simulink model "QuadRotor_PID_Simulink3d"  (R2014a)
settings: Solver=ode45  StartTime=0.0  StopTime=inf
PreLoadFcn:
  | load CommandsBus
model workspace (MAT data in the model file):
  MCOS : class17 (value not decoded)
  MCOS : class17 (value not decoded)
undefined symbols (not defined in the file or in its folder): X, Y, Z
libraries: sm_lib x829, nesl_utility x156, simulink x12, fl_lib x4, vrlib x4, aerolibtransform2 x1
(part 18 of 18)

== system QuadRotor_PID_Simulink3d/quadSimulation/Plant_Quad_Base/Quad_Yaw_Altitude/QuadRotor/P4/MotorD/Helice_1_RIGID ==
  ReferenceFrame : sm_lib/Frames and Transforms/Reference Frame  BlockFunction=simmechanics.library.frames_transforms.reference_frame
  Solid : sm_lib/Body Elements/Solid  InertiaType=Custom  Mass=0.00049709299999999999  MassUnits=kg  CenterOfMass=[0 0 -0.00012752400000000001]  CenterOfMassUnits=mm  MomentsOfInertia=[0.0011848399999999999 0.31476899999999997 0.31557499999999999]  MomentsOfInertiaUnits=kg*mm^2  ProductsOfInertia=[0 0 -7.1669699999999998e-06]  ProductsOfInertiaUnits=kg*mm^2  DensityBased=on  Density=1000  DensityUnits=kg/(m^3)  GraphicType=FromGeometry  MarkerShape=Sphere  MarkerSize=10  MarkerSizeUnits=m  GraphicVisPropType=SimpleVisualProperties  GraphicDiffuseColor=[1 1 1]  GraphicSpecularColor=[0.5 0.5 0.5 1.0]  GraphicAmbientColor=[0.15 0.15 0.15 1.0]  GraphicEmissiveColor=[0.0 0.0 0.0 1.0]  GraphicShininess=75  GraphicOpacity=1  GeometryShape=FromFile  RectangleSize=[1 1]  RectangleSizeUnits=m  BrickDimensions=[1 1 1]  BrickDimensionUnits=m  CylinderRadius=1  CylinderRadiusUnits=m  CylinderLength=1  CylinderLengthUnits=m  SphereRadius=1  SphereRadiusUnits=m  EllipsoidRadii=[1 1 1]  EllipsoidRadiiUnits=m  ExtrusionCrossSection=[1 1; -1 1; -1 -1; 1 -1]  ExtrusionCrossSectionUnits=m  ExtrusionLength=1  ExtrusionLengthUnits=m  PolygonNumSides=3  PolygonOuterRadius=1  PolygonOuterRadiusUnits=m  ExtGeomFileType=STL  ExtGeomFileName=Helice_Valor predeterminado_sldprt.STL  ExtGeomFileUnits=mm  RevolutionCrossSection=[1 1; 1 -1; 2 -1; 2 1]  RevolutionCrossSectionUnits=m  RevolutionExtent=Full  RevolutionAngle=180  RevolutionAngleUnits=deg  BlockFunction=simmechanics.library.body_elements.solid
  F : PMIOPort  Port=1  Side=Left
  connections:
  Solid/RConn1 -- ReferenceFrame/RConn1 -- F/RConn1

== system QuadRotor_PID_Simulink3d/quadSimulation/Plant_Quad_Base/Quad_Yaw_Altitude/QuadRotor/P4/MotorD/x18_11_2000kv_Micro_Brushless_1_RIGID ==
  ReferenceFrame : sm_lib/Frames and Transforms/Reference Frame  BlockFunction=simmechanics.library.frames_transforms.reference_frame
  Solid : sm_lib/Body Elements/Solid  InertiaType=Custom  Mass=10  MassUnits=g  CenterOfMass=[0 12.8438 0]  CenterOfMassUnits=mm  MomentsOfInertia=[0.43731300000000001 0.28562900000000002 0.43731300000000001]  MomentsOfInertiaUnits=kg*mm^2  ProductsOfInertia=[0 0 0]  ProductsOfInertiaUnits=kg*mm^2  DensityBased=on  Density=1000  DensityUnits=kg/(m^3)  GraphicType=FromGeometry  MarkerShape=Sphere  MarkerSize=10  MarkerSizeUnits=m  GraphicVisPropType=SimpleVisualProperties  GraphicDiffuseColor=[0.894118 0.913725 0.929412]  GraphicSpecularColor=[0.5 0.5 0.5 1.0]  GraphicAmbientColor=[0.15 0.15 0.15 1.0]  GraphicEmissiveColor=[0.0 0.0 0.0 1.0]  GraphicShininess=75  GraphicOpacity=1  GeometryShape=FromFile  RectangleSize=[1 1]  RectangleSizeUnits=m  BrickDimensions=[1 1 1]  BrickDimensionUnits=m  CylinderRadius=1  CylinderRadiusUnits=m  CylinderLength=1  CylinderLengthUnits=m  SphereRadius=1  SphereRadiusUnits=m  EllipsoidRadii=[1 1 1]  EllipsoidRadiiUnits=m  ExtrusionCrossSection=[1 1; -1 1; -1 -1; 1 -1]  ExtrusionCrossSectionUnits=m  ExtrusionLength=1  ExtrusionLengthUnits=m  PolygonNumSides=3  PolygonOuterRadius=1  PolygonOuterRadiusUnits=m  ExtGeomFileType=STL  ExtGeomFileName=18-11 2000kv Micro Brushless_Valor predeterminado_sldprt.STL  ExtGeomFileUnits=mm  RevolutionCrossSection=[1 1; 1 -1; 2 -1; 2 1]  RevolutionCrossSectionUnits=m  RevolutionExtent=Full  RevolutionAngle=180  RevolutionAngleUnits=deg  BlockFunction=simmechanics.library.body_elements.solid
  F : PMIOPort  Port=1  Side=Left
  connections:
  Solid/RConn1 -- ReferenceFrame/RConn1 -- F/RConn1

== matlab function QuadRotor_PID_Simulink3d/quadSimulation/Plant_Quad_Base/Quad_Roll_Pitch_Yaw_Altitude/QuadRotor/P2/MotorA/Thrust ==
  data: revSpeed input; Thrust output; revCnst input; revTqCnst input; Torque output
function [Thrust, Torque]  = generateThrust(revSpeed, revCnst, revTqCnst)
%#codegen
Torque = revSpeed * revTqCnst;

% Always give positive thrust (Point up)
Thrust = revCnst * revSpeed;
if (Thrust < 0)
   Thrust = Thrust * -1; 
end

== matlab function QuadRotor_PID_Simulink3d/quadSimulation/Plant_Quad_Base/Quad_Roll_Pitch_Yaw_Altitude/QuadRotor/P3/MotorC/Thrust ==
  data: revSpeed input; Thrust output; revCnst input; revTqCnst input; Torque output
function [Thrust, Torque]  = generateThrust(revSpeed, revCnst, revTqCnst)
%#codegen
Torque = revSpeed * revTqCnst;

% Always give positive thrust (Point up)
Thrust = revCnst * revSpeed;
if (Thrust < 0)
   Thrust = Thrust * -1; 
end

== matlab function QuadRotor_PID_Simulink3d/quadSimulation/Plant_Quad_Base/Quad_Roll_Pitch_Yaw_Altitude/QuadRotor/P4/MotorD/Thrust ==
  data: revSpeed input; Thrust output; revCnst input; revTqCnst input; Torque output
function [Thrust, Torque]  = generateThrust(revSpeed, revCnst, revTqCnst)
%#codegen
Torque = revSpeed * revTqCnst;

% Always give positive thrust (Point up)
Thrust = revCnst * revSpeed;
if (Thrust < 0)
   Thrust = Thrust * -1; 
end

== matlab function QuadRotor_PID_Simulink3d/quadSimulation/Plant_Quad_Base/Quad_Roll_Pitch_Yaw_Altitude/Convert/ConvertAngle ==
  data: radAngle input; AngleDeg output
function AngleDeg = getAngleDeg(radAngle)
%#codegen
AngleDeg = 0;
angleAcc = radAngle / pi;

AngleDeg = radAngle * (180/pi);
if abs(AngleDeg) > 360
    AngleDeg = mod(AngleDeg,360);
end

== matlab function QuadRotor_PID_Simulink3d/quadSimulation/Plant_Quad_Base/Quad_Roll_Pitch_Yaw_Altitude/Convert1/ConvertAngle ==
  data: radAngle input; AngleDeg output
function AngleDeg = getAngleDeg(radAngle)
%#codegen
AngleDeg = 0;
angleAcc = radAngle / pi;

AngleDeg = radAngle * (180/pi);
if abs(AngleDeg) > 360
    AngleDeg = mod(AngleDeg,360);
end

== matlab function QuadRotor_PID_Simulink3d/quadSimulation/Plant_Quad_Base/Quad_Roll_Pitch_Yaw_Altitude/Convert2/ConvertAngle ==
  data: radAngle input; AngleDeg output
function AngleDeg = getAngleDeg(radAngle)
%#codegen
AngleDeg = 0;
angleAcc = radAngle / pi;

AngleDeg = radAngle * (180/pi);
if abs(AngleDeg) > 360
    AngleDeg = mod(AngleDeg,360);
end
%AngleDeg = angleAcc * (180/pi);

== matlab function QuadRotor_PID_Simulink3d/quadSimulation/Controller/SaturateRollCmd ==
  data: spdRef input; spdOut output; inSpd input; maxVar input
function spdOut = fcn(spdRef, inSpd, maxVar)
%#codegen
minLim = -(spdRef * (maxVar/100));
maxLim = (spdRef * (maxVar/100));

spdOut = inSpd;

if inSpd > maxLim
   spdOut = maxLim;
   return;
elseif inSpd < minLim    
   spdOut = minLim; 
   return;
end

end

== matlab function QuadRotor_PID_Simulink3d/quadSimulation/Controller/SaturatePitchCmd ==
  data: spdRef input; spdOut output; inSpd input; maxVar input
function spdOut = fcn(spdRef, inSpd, maxVar)
%#codegen
minLim = -(spdRef * (maxVar/100));
maxLim = (spdRef * (maxVar/100));

spdOut = inSpd;

if inSpd > maxLim
   spdOut = maxLim;
   return;
elseif inSpd < minLim    
   spdOut = minLim; 
   return;
end

end

== matlab function QuadRotor_PID_Simulink3d/quadSimulation/Controller/SaturateRollCmd1 ==
  data: spdRef input; spdOut output; inSpd input; maxVar input
function spdOut = fcn(spdRef, inSpd, maxVar)
%#codegen
%minLim = spdRef - (spdRef * (maxVar/100));
%maxLim = spdRef + (spdRef * (maxVar/100));
minLim = -(spdRef * (maxVar/100));
maxLim = (spdRef * (maxVar/100));

spdOut = inSpd;

if inSpd > maxLim
   spdOut = maxLim;
   return;
elseif inSpd < minLim    
   spdOut = minLim; 
   return;
end

end

== matlab function QuadRotor_PID_Simulink3d/quadSimulation/Plant_Quad_Base/Quad_Altitude/Convert/ConvertAngle ==
  data: radAngle input; AngleDeg output
function AngleDeg = getAngleDeg(radAngle)
%#codegen
AngleDeg = 0;
angleAcc = radAngle / pi;

AngleDeg = radAngle * (180/pi);
if abs(AngleDeg) > 360
    AngleDeg = mod(AngleDeg,360);
end

== matlab function QuadRotor_PID_Simulink3d/quadSimulation/Plant_Quad_Base/Quad_Altitude/Convert1/ConvertAngle ==
  data: radAngle input; AngleDeg output
function AngleDeg = getAngleDeg(radAngle)
%#codegen

AngleDeg = radAngle * (180/pi);
if abs(AngleDeg) > 360
    AngleDeg = mod(AngleDeg,360);
end

== matlab function QuadRotor_PID_Simulink3d/quadSimulation/Plant_Quad_Base/Quad_Altitude/Convert2/ConvertAngle ==
  data: radAngle input; AngleDeg output
function AngleDeg = getAngleDeg(radAngle)
%#codegen
AngleDeg = 0;
angleAcc = radAngle / pi;

AngleDeg = radAngle * (180/pi);
if abs(AngleDeg) > 360
    AngleDeg = mod(AngleDeg,360);
end
%AngleDeg = angleAcc * (180/pi);

== matlab function QuadRotor_PID_Simulink3d/quadSimulation/Plant_Quad_Base/Quad_Altitude/QuadRotor/P1/MotorB/Thrust ==
  data: revSpeed input; Thrust output; revCnst input; revTqCnst input; Torque output
function [Thrust, Torque]  = generateThrust(revSpeed, revCnst, revTqCnst)
%#codegen
Torque = revSpeed * revTqCnst;

% Always give positive thrust (Point up)
Thrust = abs(revCnst * revSpeed);

== matlab function QuadRotor_PID_Simulink3d/quadSimulation/Plant_Quad_Base/Quad_Altitude/QuadRotor/P2/MotorA/Thrust ==
  data: revSpeed input; Thrust output; revCnst input; revTqCnst input; Torque output
function [Thrust, Torque]  = generateThrust(revSpeed, revCnst, revTqCnst)
%#codegen
Torque = revSpeed * revTqCnst;

% Always give positive thrust (Point up)
Thrust = revCnst * revSpeed;
if (Thrust < 0)
   Thrust = Thrust * -1; 
end

== matlab function QuadRotor_PID_Simulink3d/quadSimulation/Plant_Quad_Base/Quad_Altitude/QuadRotor/P3/MotorC/Thrust ==
  data: revSpeed input; Thrust output; revCnst input; revTqCnst input; Torque output
function [Thrust, Torque]  = generateThrust(revSpeed, revCnst, revTqCnst)
%#codegen
Torque = revSpeed * revTqCnst;

% Always give positive thrust (Point up)
Thrust = revCnst * revSpeed;
if (Thrust < 0)
   Thrust = Thrust * -1; 
end

== matlab function QuadRotor_PID_Simulink3d/quadSimulation/Plant_Quad_Base/Quad_Altitude/QuadRotor/P4/MotorD/Thrust ==
  data: revSpeed input; Thrust output; revCnst input; revTqCnst input; Torque output
function [Thrust, Torque]  = generateThrust(revSpeed, revCnst, revTqCnst)
%#codegen
Torque = revSpeed * revTqCnst;

% Always give positive thrust (Point up)
Thrust = revCnst * revSpeed;
if (Thrust < 0)
   Thrust = Thrust * -1; 
end

== matlab function QuadRotor_PID_Simulink3d/quadSimulation/Plant_Quad_Base/Quad_Pitch/Convert/ConvertAngle ==
  data: radAngle input; AngleDeg output
function AngleDeg = getAngleDeg(radAngle)
%#codegen
AngleDeg = 0;
angleAcc = radAngle / pi;

AngleDeg = radAngle * (180/pi);
if abs(AngleDeg) > 360
    AngleDeg = mod(AngleDeg,360);
end

== matlab function QuadRotor_PID_Simulink3d/quadSimulation/Plant_Quad_Base/Quad_Pitch/Convert1/ConvertAngle ==
  data: radAngle input; AngleDeg output
function AngleDeg = getAngleDeg(radAngle)
%#codegen
AngleDeg = 0;
angleAcc = radAngle / pi;

AngleDeg = radAngle * (180/pi);
if abs(AngleDeg) > 360
    AngleDeg = mod(AngleDeg,360);
end

== matlab function QuadRotor_PID_Simulink3d/quadSimulation/Plant_Quad_Base/Quad_Pitch/Convert2/ConvertAngle ==
  data: radAngle input; AngleDeg output
function AngleDeg = getAngleDeg(radAngle)
%#codegen
AngleDeg = 0;
angleAcc = radAngle / pi;

AngleDeg = radAngle * (180/pi);
if abs(AngleDeg) > 360
    AngleDeg = mod(AngleDeg,360);
end
%AngleDeg = angleAcc * (180/pi);

== matlab function QuadRotor_PID_Simulink3d/quadSimulation/Plant_Quad_Base/Quad_Pitch/QuadRotor/P1/MotorB/Thrust ==
  data: revSpeed input; Thrust output; revCnst input; revTqCnst input; Torque output
function [Thrust, Torque]  = generateThrust(revSpeed, revCnst, revTqCnst)
%#codegen
Torque = revSpeed * revTqCnst;

% Always give positive thrust (Point up)
Thrust = abs(revCnst * revSpeed);

== matlab function QuadRotor_PID_Simulink3d/quadSimulation/Plant_Quad_Base/Quad_Pitch/QuadRotor/P2/MotorA/Thrust ==
  data: revSpeed input; Thrust output; revCnst input; revTqCnst input; Torque output
function [Thrust, Torque]  = generateThrust(revSpeed, revCnst, revTqCnst)
%#codegen
Torque = revSpeed * revTqCnst;

% Always give positive thrust (Point up)
Thrust = revCnst * revSpeed;
if (Thrust < 0)
   Thrust = Thrust * -1; 
end

== matlab function QuadRotor_PID_Simulink3d/quadSimulation/Plant_Quad_Base/Quad_Pitch/QuadRotor/P3/MotorC/Thrust ==
  data: revSpeed input; Thrust output; revCnst input; revTqCnst input; Torque output
function [Thrust, Torque]  = generateThrust(revSpeed, revCnst, revTqCnst)
%#codegen
Torque = revSpeed * revTqCnst;

% Always give positive thrust (Point up)
Thrust = revCnst * revSpeed;
if (Thrust < 0)
   Thrust = Thrust * -1; 
end

== matlab function QuadRotor_PID_Simulink3d/quadSimulation/Plant_Quad_Base/Quad_Pitch/QuadRotor/P4/MotorD/Thrust ==
  data: revSpeed input; Thrust output; revCnst input; revTqCnst input; Torque output
function [Thrust, Torque]  = generateThrust(revSpeed, revCnst, revTqCnst)
%#codegen
Torque = revSpeed * revTqCnst;

% Always give positive thrust (Point up)
Thrust = revCnst * revSpeed;
if (Thrust < 0)
   Thrust = Thrust * -1; 
end

== matlab function QuadRotor_PID_Simulink3d/quadSimulation/Plant_Quad_Base/Quad_Yaw/Convert/ConvertAngle ==
  data: radAngle input; AngleDeg output
function AngleDeg = getAngleDeg(radAngle)
%#codegen
AngleDeg = 0;
angleAcc = radAngle / pi;

AngleDeg = radAngle * (180/pi);
if abs(AngleDeg) > 360
    AngleDeg = mod(AngleDeg,360);
end

== matlab function QuadRotor_PID_Simulink3d/quadSimulation/Plant_Quad_Base/Quad_Yaw/Convert1/ConvertAngle ==
  data: radAngle input; AngleDeg output
function AngleDeg = getAngleDeg(radAngle)
%#codegen
AngleDeg = 0;
angleAcc = radAngle / pi;

AngleDeg = radAngle * (180/pi);
if abs(AngleDeg) > 360
    AngleDeg = mod(AngleDeg,360);
end

== matlab function QuadRotor_PID_Simulink3d/quadSimulation/Plant_Quad_Base/Quad_Yaw/Convert2/ConvertAngle ==
  data: radAngle input; AngleDeg output
function AngleDeg = getAngleDeg(radAngle)
%#codegen
AngleDeg = 0;
angleAcc = radAngle / pi;

AngleDeg = radAngle * (180/pi);
if abs(AngleDeg) > 360
    AngleDeg = mod(AngleDeg,360);
end
%AngleDeg = angleAcc * (180/pi);

== matlab function QuadRotor_PID_Simulink3d/quadSimulation/Plant_Quad_Base/Quad_Yaw/QuadRotor/P1/MotorB/Thrust ==
  data: revSpeed input; Thrust output; revCnst input; revTqCnst input; Torque output
function [Thrust, Torque]  = generateThrust(revSpeed, revCnst, revTqCnst)
%#codegen
Torque = revSpeed * revTqCnst;

% Always give positive thrust (Point up)
Thrust = abs(revCnst * revSpeed);

== matlab function QuadRotor_PID_Simulink3d/quadSimulation/Plant_Quad_Base/Quad_Yaw/QuadRotor/P2/MotorA/Thrust ==
  data: revSpeed input; Thrust output; revCnst input; revTqCnst input; Torque output
function [Thrust, Torque]  = generateThrust(revSpeed, revCnst, revTqCnst)
%#codegen
Torque = revSpeed * revTqCnst;

% Always give positive thrust (Point up)
Thrust = revCnst * revSpeed;
if (Thrust < 0)
   Thrust = Thrust * -1; 
end

== matlab function QuadRotor_PID_Simulink3d/quadSimulation/Plant_Quad_Base/Quad_Yaw/QuadRotor/P3/MotorC/Thrust ==
  data: revSpeed input; Thrust output; revCnst input; revTqCnst input; Torque output
function [Thrust, Torque]  = generateThrust(revSpeed, revCnst, revTqCnst)
%#codegen
Torque = revSpeed * revTqCnst;

% Always give positive thrust (Point up)
Thrust = revCnst * revSpeed;
if (Thrust < 0)
   Thrust = Thrust * -1; 
end

== matlab function QuadRotor_PID_Simulink3d/quadSimulation/Plant_Quad_Base/Quad_Yaw/QuadRotor/P4/MotorD/Thrust ==
  data: revSpeed input; Thrust output; revCnst input; revTqCnst input; Torque output
function [Thrust, Torque]  = generateThrust(revSpeed, revCnst, revTqCnst)
%#codegen
Torque = revSpeed * revTqCnst;

% Always give positive thrust (Point up)
Thrust = revCnst * revSpeed;
if (Thrust < 0)
   Thrust = Thrust * -1; 
end

== matlab function QuadRotor_PID_Simulink3d/quadSimulation/Plant_Quad_Base/Quad_Roll/Convert/ConvertAngle ==
  data: radAngle input; AngleDeg output
function AngleDeg = getAngleDeg(radAngle)
%#codegen
AngleDeg = 0;
angleAcc = radAngle / pi;

AngleDeg = radAngle * (180/pi);
if abs(AngleDeg) > 360
    AngleDeg = mod(AngleDeg,360);
end

== matlab function QuadRotor_PID_Simulink3d/quadSimulation/Plant_Quad_Base/Quad_Roll/Convert1/ConvertAngle ==
  data: radAngle input; AngleDeg output
function AngleDeg = getAngleDeg(radAngle)
%#codegen
AngleDeg = 0;
angleAcc = radAngle / pi;

AngleDeg = radAngle * (180/pi);
if abs(AngleDeg) > 360
    AngleDeg = mod(AngleDeg,360);
end

== matlab function QuadRotor_PID_Simulink3d/quadSimulation/Plant_Quad_Base/Quad_Roll/Convert2/ConvertAngle ==
  data: radAngle input; AngleDeg output
function AngleDeg = getAngleDeg(radAngle)
%#codegen
AngleDeg = 0;
angleAcc = radAngle / pi;

AngleDeg = radAngle * (180/pi);
if abs(AngleDeg) > 360
    AngleDeg = mod(AngleDeg,360);
end
%AngleDeg = angleAcc * (180/pi);

== matlab function QuadRotor_PID_Simulink3d/quadSimulation/Plant_Quad_Base/Quad_Roll/QuadRotor/P1/MotorB/Thrust ==
  data: revSpeed input; Thrust output; revCnst input; revTqCnst input; Torque output
function [Thrust, Torque]  = generateThrust(revSpeed, revCnst, revTqCnst)
%#codegen
Torque = revSpeed * revTqCnst;

% Always give positive thrust (Point up)
Thrust = abs(revCnst * revSpeed);

== matlab function QuadRotor_PID_Simulink3d/quadSimulation/Plant_Quad_Base/Quad_Roll/QuadRotor/P2/MotorA/Thrust ==
  data: revSpeed input; Thrust output; revCnst input; revTqCnst input; Torque output
function [Thrust, Torque]  = generateThrust(revSpeed, revCnst, revTqCnst)
%#codegen
Torque = revSpeed * revTqCnst;

% Always give positive thrust (Point up)
Thrust = revCnst * revSpeed;
if (Thrust < 0)
   Thrust = Thrust * -1; 
end

== matlab function QuadRotor_PID_Simulink3d/quadSimulation/Plant_Quad_Base/Quad_Roll_Pitch_Yaw_Altitude/QuadRotor/P1/MotorB/Thrust ==
  data: revSpeed input; Thrust output; revCnst input; revTqCnst input; Torque output
function [Thrust, Torque]  = generateThrust(revSpeed, revCnst, revTqCnst)
%#codegen
Torque = revSpeed * revTqCnst;

% Always give positive thrust (Point up)
Thrust = abs(revCnst * revSpeed);

== matlab function QuadRotor_PID_Simulink3d/quadSimulation/Plant_Quad_Base/Quad_Roll/QuadRotor/P3/MotorC/Thrust ==
  data: revSpeed input; Thrust output; revCnst input; revTqCnst input; Torque output
function [Thrust, Torque]  = generateThrust(revSpeed, revCnst, revTqCnst)
%#codegen
Torque = revSpeed * revTqCnst;

% Always give positive thrust (Point up)
Thrust = revCnst * revSpeed;
if (Thrust < 0)
   Thrust = Thrust * -1; 
end

== matlab function QuadRotor_PID_Simulink3d/quadSimulation/Plant_Quad_Base/Quad_Roll/QuadRotor/P4/MotorD/Thrust ==
  data: revSpeed input; Thrust output; revCnst input; revTqCnst input; Torque output
function [Thrust, Torque]  = generateThrust(revSpeed, revCnst, revTqCnst)
%#codegen
Torque = revSpeed * revTqCnst;

% Always give positive thrust (Point up)
Thrust = revCnst * revSpeed;
if (Thrust < 0)
   Thrust = Thrust * -1; 
end

== matlab function QuadRotor_PID_Simulink3d/quadSimulation/Plant_Quad_Base/Quad_Roll_Pitch_Yaw/Convert/ConvertAngle ==
  data: radAngle input; AngleDeg output
function AngleDeg = getAngleDeg(radAngle)
%#codegen
AngleDeg = 0;
angleAcc = radAngle / pi;

AngleDeg = radAngle * (180/pi);
if abs(AngleDeg) > 360
    AngleDeg = mod(AngleDeg,360);
end

== matlab function QuadRotor_PID_Simulink3d/quadSimulation/Plant_Quad_Base/Quad_Roll_Pitch_Yaw/Convert1/ConvertAngle ==
  data: radAngle input; AngleDeg output
function AngleDeg = getAngleDeg(radAngle)
%#codegen
AngleDeg = 0;
angleAcc = radAngle / pi;

AngleDeg = radAngle * (180/pi);
if abs(AngleDeg) > 360
    AngleDeg = mod(AngleDeg,360);
end

== matlab function QuadRotor_PID_Simulink3d/quadSimulation/Plant_Quad_Base/Quad_Roll_Pitch_Yaw/Convert2/ConvertAngle ==
  data: radAngle input; AngleDeg output
function AngleDeg = getAngleDeg(radAngle)
%#codegen
AngleDeg = 0;
angleAcc = radAngle / pi;

AngleDeg = radAngle * (180/pi);
if abs(AngleDeg) > 360
    AngleDeg = mod(AngleDeg,360);
end
%AngleDeg = angleAcc * (180/pi);

== matlab function QuadRotor_PID_Simulink3d/quadSimulation/Plant_Quad_Base/Quad_Roll_Pitch_Yaw/QuadRotor/P1/MotorB/Thrust ==
  data: revSpeed input; Thrust output; revCnst input; revTqCnst input; Torque output
function [Thrust, Torque]  = generateThrust(revSpeed, revCnst, revTqCnst)
%#codegen
Torque = revSpeed * revTqCnst;

% Always give positive thrust (Point up)
Thrust = abs(revCnst * revSpeed);

== matlab function QuadRotor_PID_Simulink3d/quadSimulation/Plant_Quad_Base/Quad_Roll_Pitch_Yaw/QuadRotor/P2/MotorA/Thrust ==
  data: revSpeed input; Thrust output; revCnst input; revTqCnst input; Torque output
function [Thrust, Torque]  = generateThrust(revSpeed, revCnst, revTqCnst)
%#codegen
Torque = revSpeed * revTqCnst;

% Always give positive thrust (Point up)
Thrust = revCnst * revSpeed;
if (Thrust < 0)
   Thrust = Thrust * -1; 
end

== matlab function QuadRotor_PID_Simulink3d/quadSimulation/Plant_Quad_Base/Quad_Roll_Pitch_Yaw/QuadRotor/P3/MotorC/Thrust ==
  data: revSpeed input; Thrust output; revCnst input; revTqCnst input; Torque output
function [Thrust, Torque]  = generateThrust(revSpeed, revCnst, revTqCnst)
%#codegen
Torque = revSpeed * revTqCnst;

% Always give positive thrust (Point up)
Thrust = revCnst * revSpeed;
if (Thrust < 0)
   Thrust = Thrust * -1; 
end

== matlab function QuadRotor_PID_Simulink3d/quadSimulation/Plant_Quad_Base/Quad_Roll_Pitch_Yaw/QuadRotor/P4/MotorD/Thrust ==
  data: revSpeed input; Thrust output; revCnst input; revTqCnst input; Torque output
function [Thrust, Torque]  = generateThrust(revSpeed, revCnst, revTqCnst)
%#codegen
Torque = revSpeed * revTqCnst;

% Always give positive thrust (Point up)
Thrust = revCnst * revSpeed;
if (Thrust < 0)
   Thrust = Thrust * -1; 
end

== matlab function QuadRotor_PID_Simulink3d/quadSimulation/Plant_Quad_Base/Quad_Yaw_Altitude/Convert/ConvertAngle ==
  data: radAngle input; AngleDeg output
function AngleDeg = getAngleDeg(radAngle)
%#codegen
AngleDeg = 0;
angleAcc = radAngle / pi;

AngleDeg = radAngle * (180/pi);
if abs(AngleDeg) > 360
    AngleDeg = mod(AngleDeg,360);
end

== matlab function QuadRotor_PID_Simulink3d/quadSimulation/Plant_Quad_Base/Quad_Yaw_Altitude/Convert1/ConvertAngle ==
  data: radAngle input; AngleDeg output
function AngleDeg = getAngleDeg(radAngle)
%#codegen
AngleDeg = 0;
angleAcc = radAngle / pi;

AngleDeg = radAngle * (180/pi);
if abs(AngleDeg) > 360
    AngleDeg = mod(AngleDeg,360);
end

== matlab function QuadRotor_PID_Simulink3d/quadSimulation/Plant_Quad_Base/Quad_Yaw_Altitude/Convert2/ConvertAngle ==
  data: radAngle input; AngleDeg output
function AngleDeg = getAngleDeg(radAngle)
%#codegen
AngleDeg = 0;
angleAcc = radAngle / pi;

AngleDeg = radAngle * (180/pi);
if abs(AngleDeg) > 360
    AngleDeg = mod(AngleDeg,360);
end
%AngleDeg = angleAcc * (180/pi);

== matlab function QuadRotor_PID_Simulink3d/quadSimulation/Plant_Quad_Base/Quad_Yaw_Altitude/QuadRotor/P1/MotorB/Thrust ==
  data: revSpeed input; Thrust output; revCnst input; revTqCnst input; Torque output
function [Thrust, Torque]  = generateThrust(revSpeed, revCnst, revTqCnst)
%#codegen
Torque = revSpeed * revTqCnst;

% Always give positive thrust (Point up)
Thrust = abs(revCnst * revSpeed);

== matlab function QuadRotor_PID_Simulink3d/quadSimulation/Plant_Quad_Base/Quad_Yaw_Altitude/QuadRotor/P2/MotorA/Thrust ==
  data: revSpeed input; Thrust output; revCnst input; revTqCnst input; Torque output
function [Thrust, Torque]  = generateThrust(revSpeed, revCnst, revTqCnst)
%#codegen
Torque = revSpeed * revTqCnst;

% Always give positive thrust (Point up)
Thrust = revCnst * revSpeed;
if (Thrust < 0)
   Thrust = Thrust * -1; 
end

== matlab function QuadRotor_PID_Simulink3d/quadSimulation/Plant_Quad_Base/Quad_Yaw_Altitude/QuadRotor/P3/MotorC/Thrust ==
  data: revSpeed input; Thrust output; revCnst input; revTqCnst input; Torque output
function [Thrust, Torque]  = generateThrust(revSpeed, revCnst, revTqCnst)
%#codegen
Torque = revSpeed * revTqCnst;

% Always give positive thrust (Point up)
Thrust = revCnst * revSpeed;
if (Thrust < 0)
   Thrust = Thrust * -1; 
end

== matlab function QuadRotor_PID_Simulink3d/quadSimulation/Plant_Quad_Base/Quad_Yaw_Altitude/QuadRotor/P4/MotorD/Thrust ==
  data: revSpeed input; Thrust output; revCnst input; revTqCnst input; Torque output
function [Thrust, Torque]  = generateThrust(revSpeed, revCnst, revTqCnst)
%#codegen
Torque = revSpeed * revTqCnst;

% Always give positive thrust (Point up)
Thrust = revCnst * revSpeed;
if (Thrust < 0)
   Thrust = Thrust * -1; 
end

== matlab function QuadRotor_PID_Simulink3d/quadSimulation/Plant_Quad_Base/Quad_6Dof/Convert/ConvertAngle ==
  data: radAngle input; AngleDeg output
function AngleDeg = getAngleDeg(radAngle)
%#codegen
AngleDeg = 0;
angleAcc = radAngle / pi;

AngleDeg = radAngle * (180/pi);
if abs(AngleDeg) > 360
    AngleDeg = mod(AngleDeg,360);
end

== matlab function QuadRotor_PID_Simulink3d/quadSimulation/Plant_Quad_Base/Quad_6Dof/Convert1/ConvertAngle ==
  data: radAngle input; AngleDeg output
function AngleDeg = getAngleDeg(radAngle)
%#codegen
AngleDeg = 0;
angleAcc = radAngle / pi;

AngleDeg = radAngle * (180/pi);
if abs(AngleDeg) > 360
    AngleDeg = mod(AngleDeg,360);
end

== matlab function QuadRotor_PID_Simulink3d/quadSimulation/Plant_Quad_Base/Quad_6Dof/Convert2/ConvertAngle ==
  data: radAngle input; AngleDeg output
function AngleDeg = getAngleDeg(radAngle)
%#codegen
AngleDeg = 0;
angleAcc = radAngle / pi;

AngleDeg = radAngle * (180/pi);
if abs(AngleDeg) > 360
    AngleDeg = mod(AngleDeg,360);
end
%AngleDeg = angleAcc * (180/pi);

== matlab function QuadRotor_PID_Simulink3d/quadSimulation/Plant_Quad_Base/Quad_6Dof/QuadRotor/P1/MotorB/Thrust ==
  data: revSpeed input; Thrust output; revCnst input; revTqCnst input; Torque output
function [Thrust, Torque]  = generateThrust(revSpeed, revCnst, revTqCnst)
%#codegen
Torque = revSpeed * revTqCnst;

% Always give positive thrust (Point up)
Thrust = abs(revCnst * revSpeed);

== matlab function QuadRotor_PID_Simulink3d/quadSimulation/Plant_Quad_Base/Quad_6Dof/QuadRotor/P2/MotorA/Thrust ==
  data: revSpeed input; Thrust output; revCnst input; revTqCnst input; Torque output
function [Thrust, Torque]  = generateThrust(revSpeed, revCnst, revTqCnst)
%#codegen
Torque = revSpeed * revTqCnst;

% Always give positive thrust (Point up)
Thrust = revCnst * revSpeed;
if (Thrust < 0)
   Thrust = Thrust * -1; 
end

== matlab function QuadRotor_PID_Simulink3d/quadSimulation/Plant_Quad_Base/Quad_6Dof/QuadRotor/P3/MotorC/Thrust ==
  data: revSpeed input; Thrust output; revCnst input; revTqCnst input; Torque output
function [Thrust, Torque]  = generateThrust(revSpeed, revCnst, revTqCnst)
%#codegen
Torque = revSpeed * revTqCnst;

% Always give positive thrust (Point up)
Thrust = revCnst * revSpeed;
if (Thrust < 0)
   Thrust = Thrust * -1; 
end

== matlab function QuadRotor_PID_Simulink3d/quadSimulation/Plant_Quad_Base/Quad_6Dof/QuadRotor/P4/MotorD/Thrust ==
  data: revSpeed input; Thrust output; revCnst input; revTqCnst input; Torque output
function [Thrust, Torque]  = generateThrust(revSpeed, revCnst, revTqCnst)
%#codegen
Torque = revSpeed * revTqCnst;

% Always give positive thrust (Point up)
Thrust = revCnst * revSpeed;
if (Thrust < 0)
   Thrust = Thrust * -1; 
end

== stateflow chart QuadRotor_PID_Simulink3d/Chart ==
  state FailSaves [parallel]
    settings: executionOrder=2
  state mainLoop [parallel]
    settings: executionOrder=1
    note: wait for 5 heartBeats
    note: request streams one  by one,
        | if data  not received after
        | 1 sec- request again
    note: TODO dont arm if throttle on
    state Sky
      state Autonomous
        entry:
        during:
        %if controlCommands.RPTYUp
        commandsOut=controlCommands;
        %end
        exit:
      state Manual
        during:
        commandsOut=joystickInput;
      Manual -> Autonomous : [joystickInput.nav]
      (default) -> Manual
      Autonomous -> Manual : [~joystickInput.nav]
    (default) -> Sky
  data: data function_output; length function_output; streamId function_input; data function_output; length function_output; armdisarm function_input; data function_output; length function_output; R function_input; P function_input; T function_input; Y function_input; joystickInput input Bus: CommandsBus size=1; controlCommands input Bus: CommandsBus size=1; commandsOut output Bus: CommandsBus
  events: sendme output FUNCTION_CALL_EVENT
  function [data,length] = requestStreams(streamId):
    | function  [data,length] = requestStreams(streamId)
    | data2 = zeros(256,1,'uint8');
    | length =uint8(0);
    | data=data2;
    | if ~coder.target('SFun')
    |   length=coder.ceval('requestStream', coder.ref(data2),uint8(streamId));
    | 
    |   
    |   data=data2;
    | end
  function [data,length] = sendArmDisarmFun(armdisarm):
    | function  [data,length] = sendArmDisarmFun(armdisarm)
    | data2 = zeros(256,1,'uint8');
    | length =uint8(0);
    | data=data2;
    | if ~coder.target('SFun')
    |   length=coder.ceval('sendArmDisarm', coder.ref(data2),uint8(armdisarm));
    |   data=data2;  
    | end
  function [data,length] = sendRPTY(R, P, T,Y):
    | function [data,length] = sendRPTY(R, P, T,Y)
    | data2 = zeros(256,1,'uint8');
    | length =uint8(0);
    | data=data2;
    | if ~coder.target('SFun')
    |     length=coder.ceval('sendRPTY',...
    |         coder.ref(data2),uint16(R),uint16(P),uint16(T),uint16(Y));
    |     data=data2;
    | end
